simulink model "control_loop"  (R2023b)
settings: Solver=ode45  StartTime=0.0  StopTime=250  RelTol=1e-3
values from neighbouring files (symbols this model uses):
  alfa1 = 40    [vehicle_params.m]
  alfa2 = 35    [vehicle_params.m]
  alfa3 = 16    [vehicle_params.m]
  alfa4 = 12    [vehicle_params.m]
  alfa5 = 10    [vehicle_params.m]
  m = 1200    [vehicle_params.m]
libraries: slpidlib x1
(part 1 of 3)
settings Model: Creator=luigivanacore  LastModifiedBy=luigivanacore

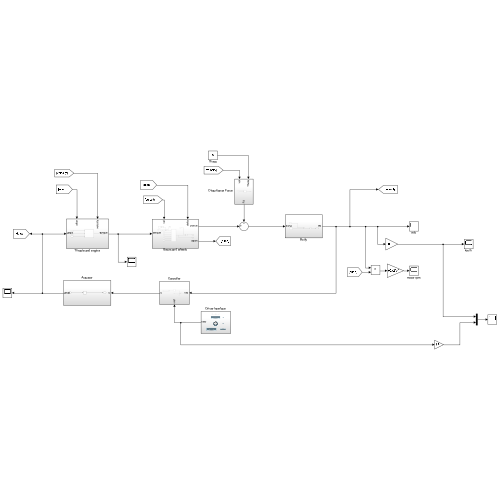
[thumbnail: Simulink's stored preview of the top-level diagram]
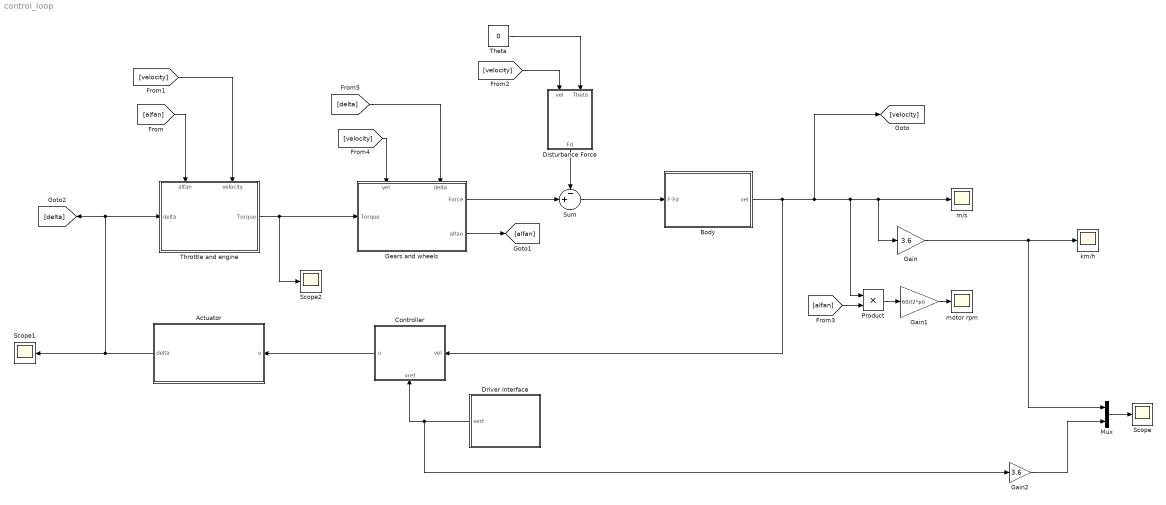
== system control_loop ==
  Actuator : Subsystem
  Body : Subsystem
  Controller : Subsystem
      settings: PortSchema="{\"entries\":[{\"content\":{\"sides\":[{\"content\":{\"connectorIds\":[\"In1\"]},\"type\":\"ConnectorPlacement.EquallySpacedRectSide\",\"uuid\":\"815a8116-67e3-4a02-82b8-981e60629451\"},{\"content\":{\"connectorIds\":[\"Out1\"],\"side\":\"RIGHT\"},\"type\":\"ConnectorPlacement.EquallySpacedRectSide\",\"uuid\":\"1dae2179-9fb3-4c97-8f3b-f0bd153ebc00\"},{\"content\":{\"side\":\"TOP\"},\"type\":\"ConnectorPlacement.EquallySpacedRectSide\",\"uuid\":\"4e651af0-7914-4384-8a44-3b25a5cc1452\"},{\"content\":{\"connectorIds\":[\"In2\"],\"side\":\"BOTTOM\"},\"type\":\"ConnectorPlacement.EquallySpacedRectSide\",\"uuid\":\"f62a5d4a-e183-4c96-8c62-4d382a034d6e\"}]},\"type\":\"ConnectorPlacement.EquallySpacedConnector\",\"uuid\":\"94ef7d1f-8223-43e7-abe2-faa3828e716d\"}],\"packageUris\":[\"http://schema.mathworks.com/mf0/Connector/R2020b\"],\"version\":\"1.0\"}"
  Disturbance Force : Subsystem
  Driver Interface : Subsystem
  Gain : Gain  Gain=3.6
  Gain1 : Gain  Gain=60/(2*pi)
  Gain2 : Gain  Gain=3.6
  Gears and wheels : Subsystem
      settings: PortSchema="{\"entries\":[{\"content\":{\"sides\":[{\"content\":{\"connectorIds\":[\"In1\"]},\"type\":\"ConnectorPlacement.EquallySpacedRectSide\",\"uuid\":\"f01132aa-ae65-48b1-9593-a40f4dadf77d\"},{\"content\":{\"connectorIds\":[\"Out1\",\"Out2\"],\"side\":\"RIGHT\"},\"type\":\"ConnectorPlacement.EquallySpacedRectSide\",\"uuid\":\"e47514dc-ddd4-444e-83cf-5b671ddd4ef4\"},{\"content\":{\"connectorIds\":[\"In2\",\"In3\"],\"side\":\"TOP\"},\"type\":\"ConnectorPlacement.EquallySpacedRectSide\",\"uuid\":\"663b35f1-4f75-45cc-9ed8-a4d7f9da6290\"}]},\"type\":\"ConnectorPlacement.EquallySpacedConnector\",\"uuid\":\"3cab4af6-754f-455e-8d1f-e46628c9ca75\"}],\"packageUris\":[\"http://schema.mathworks.com/mf0/Connector/R2020b\"],\"version\":\"1.0\"}"
  Mux : Mux  Inputs=2
  Product : Product
  Scope : Scope
  Scope1 : Scope
  Scope2 : Scope
  Sum : Sum  Inputs=-+|
  Theta : Constant  Value=0
  Throttle and engine : Subsystem
      settings: PortSchema="{\"entries\":[{\"content\":{\"sides\":[{\"content\":{\"connectorIds\":[\"In1\"]},\"type\":\"ConnectorPlacement.EquallySpacedRectSide\",\"uuid\":\"397f244c-8194-4aef-8985-f671201af3c3\"},{\"content\":{\"connectorIds\":[\"Out1\"],\"side\":\"RIGHT\"},\"type\":\"ConnectorPlacement.EquallySpacedRectSide\",\"uuid\":\"9f5999d7-4a95-4dff-848c-9e50ba67840b\"},{\"content\":{\"connectorIds\":[\"In2\",\"In3\"],\"side\":\"TOP\"},\"type\":\"ConnectorPlacement.EquallySpacedRectSide\",\"uuid\":\"681c96c1-fec8-4989-9d1c-1b7bb5ffba79\"}]},\"type\":\"ConnectorPlacement.EquallySpacedConnector\",\"uuid\":\"737cb2cd-e536-400e-93b2-7fb809a23c8e\"}],\"packageUris\":[\"http://schema.mathworks.com/mf0/Connector/R2020b\"],\"version\":\"1.0\"}"
  km/h : Scope
  m/s : Scope
  motor rpm : Scope
  wires:
  Theta/1 -> Disturbance Force/2(Theta)
  Disturbance Force/1(Fd) -> Sum/1
  Sum/1 -> Body/1(F-Fd)
  [alfan] -> Throttle and engine/2(alfan)
  Actuator/1(delta) -> Scope1/1, [delta], Throttle and engine/1(delta)
  [velocity] -> Disturbance Force/1(vel)
  Throttle and engine/1(Torque) -> Gears and wheels/1(Torque), Scope2/1
  [velocity] -> Throttle and engine/3(velocity)
  Controller/1(u) -> Actuator/1(u)
  Body/1(vel) -> Controller/1(vel), [velocity], Product/1, Gain/1, m/s/1
  Gain/1 -> Mux/1, km/h/1
  [alfan] -> Product/2
  Gain1/1 -> motor rpm/1
  Product/1 -> Gain1/1
  [velocity] -> Gears and wheels/2(vel)
  Gears and wheels/2(alfan) -> [alfan]
  Gears and wheels/1(Force) -> Sum/2
  [delta] -> Gears and wheels/3(delta)
  Driver Interface/1(verf) -> Gain2/1, Controller/2(vref)
  Mux/1 -> Scope/1
  Gain2/1 -> Mux/2

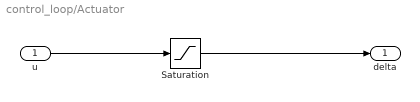
== system control_loop/Actuator ==
  u : Inport
  Saturation : Saturate  UpperLimit=1  LowerLimit=0
  delta : Outport
  wires:
  Saturation/1 -> delta/1
  u/1 -> Saturation/1

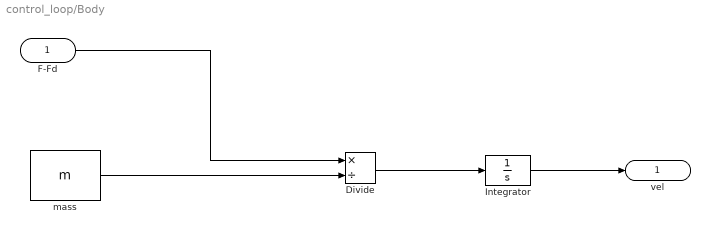
== system control_loop/Body ==
  F-Fd : Inport
  Divide : Product  Inputs=*/
  Integrator : Integrator
  mass : Constant  Value=m
  vel : Outport
  wires:
  mass/1 -> Divide/2
  F-Fd/1 -> Divide/1
  Divide/1 -> Integrator/1
  Integrator/1 -> vel/1

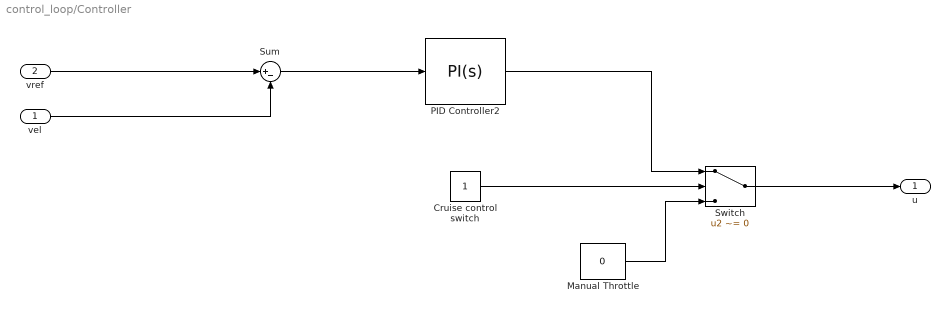
== system control_loop/Controller ==
  vel : Inport
  vref : Inport  Port=2
  Cruise control switch : Constant
  Manual Throttle : Constant  Value=0
  PID Controller2 : slpidlib/PID Controller  Controller=PI  Form=Parallel  TimeDomain=Continuous-time  UseExternalTs=off  SampleTime=-1  IntegratorMethod=Forward Euler  FilterMethod=Forward Euler  ControllerParametersSource=internal  P=1.8  I=0.7  UseKiTs=on  D=0  N=100  UseFilter=on  TunerSelectOption=Transfer Function Based (PID Tuner App)  InitialConditionSource=internal  InitialConditionForIntegrator=0  InitialConditionForFilter=0  DifferentiatorICPrevScaledInput=0  ExternalReset=none  TrackingMode=off  Kt=1  LimitOutput=on  SatLimitsSource=internal  UpperSaturationLimit=1  LowerSaturationLimit=0  LinearizeAsGain=on  AntiWindupMode=clamping  Kb=1  LimitIntegrator=off  UpperIntegratorSaturationLimit=inf  LowerIntegratorSaturationLimit=-inf  POutMin=[]  POutMax=[]  IOutMin=[]  IOutMax=[]  DOutMin=[]  DOutMax=[]  NOutMin=[]  NOutMax=[]  SumOutMin=[]  SumOutMax=[]  SaturationOutMin=[]  SaturationOutMax=[]  PParamMin=[]  PParamMax=[]  IParamMin=[]  IParamMax=[]  DParamMin=[]  DParamMax=[]  NParamMin=[]  NParamMax=[]  KbParamMin=[]  KbParamMax=[]  KtParamMin=[]  KtParamMax=[]  KbOutMin=[]  KbOutMax=[]  KtOutMin=[]  KtOutMax=[]  IntegratorOutMin=[]  IntegratorOutMax=[]  FilterOutMin=[]  FilterOutMax=[]  SumI1OutMin=[]  SumI1OutMax=[]  SumI2OutMin=[]  SumI2OutMax=[]  SumI3OutMin=[]  SumI3OutMax=[]  SumI4OutMin=[]  SumI4OutMax=[]  SumDOutMin=[]  SumDOutMax=[]  DifferentiatorOutMin=[]  DifferentiatorOutMax=[]  FilterDiffOutCoefMin=[]  FilterDiffOutCoefMax=[]  ReciprocalOutMin=[]  ReciprocalOutMax=[]  SumDenOutMin=[]  SumDenOutMax=[]  SumNumOutMin=[]  SumNumOutMax=[]  DivideOutMin=[]  DivideOutMax=[]  UdiffTsProdOutMin=[]  UdiffTsProdOutMax=[]  NTsProdOutMin=[]  NTsProdOutMax=[]  UintegralTsProdOutMin=[]  UintegralTsProdOutMax=[]  UngainTsProdOutMin=[]  UngainTsProdOutMax=[]  ClampingZeroOutDataTypeStr=Inherit: Inherit via back propagation  ClampingZeroOutMin=[]  ClampingZeroOutMax=[]  FilterDenConstantOutDataTypeStr=Inherit: Inherit via back propagation  FilterDenConstantOutMin=[]  FilterDenConstantOutMax=[]  PCopyOutDataTypeStr=Inherit: Inherit via back propagation  PCopyOutMin=[]  PCopyOutMax=[]  NCopyOutDataTypeStr=Inherit: Inherit via back propagation  NCopyOutMin=[]  NCopyOutMax=[]  IntegratorContinuousStateAttributes=''  IntegratorStateMustResolveToSignalObject=off  IntegratorRTWStateStorageClass=Auto  FilterContinuousStateAttributes=''  FilterStateMustResolveToSignalObject=off  FilterRTWStateStorageClass=Auto  ParallelPVariant=InternalParameters  IdealPVariant=Disabled  IVariant=InternalParameters  DVariant=Disabled  IntegratorVariant=Continuous  SatVariant=Enabled  AWVariant=ContClampingParallel  PCopyVariant=Disabled  TRVariant=Disabled  FdbkBlocksVariant=Forward  IdealPFdbkVariant=Disabled  SatFdbkVariant=Disabled  DerivativeFilterVariant=Disabled  NVariant=Disabled  NCopyVariant=Disabled_SignalSpec  FilterICVariant=Disabled  IntegratorICVariant=InternalICs  ExternalResetVariant=Disabled  TRSumVariant=Passthrough  SumFdbkVariant=Disabled  SumVariant=Sum_PI  TsampFilterVariant=InternalTs  TsampNgainVariant=Passthrough  TsampIntegralVariant=Disabled_SignalSpec  ExternalSaturationOutDataTypeStr=Inherit: Same as second input
  Sum : Sum  Inputs=|+-
  Switch : Switch  Criteria=u2 ~= 0  Threshold=0.5  SaturateOnIntegerOverflow=off  InputSameDT=off
  u : Outport
  wires:
  vref/1 -> Sum/1
  vel/1 -> Sum/2
  Sum/1 -> PID Controller2/1
  Switch/1 -> u/1
  Cruise control switch/1 -> Switch/2
  Manual Throttle/1 -> Switch/3
  PID Controller2/1 -> Switch/1

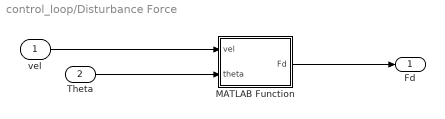
== system control_loop/Disturbance Force ==
  vel : Inport
  Theta : Inport  Port=2
  MATLAB Function : MATLAB Function  TreatAsAtomicUnit=on
  Fd : Outport
  wires:
  MATLAB Function/1(Fd) -> Fd/1
  vel/1 -> MATLAB Function/1(vel)
  Theta/1 -> MATLAB Function/2(theta)
